simulink model "SIMU4INDIFullLoop"  (R2021a)
settings: Solver=VariableStepAuto  StartTime=0.0  StopTime=40  RelTol=1e-3
values from neighbouring files (symbols this model uses):
  Ahg2 = blkdiag(Ahg2, Ahcg)    [HinFSynINDIFullLoop.m]
  Ahs3 = blkdiag(Ahs3, Ahcs)    [HinFSynINDIFullLoop.m]
  Ahs7 = blkdiag(Ahs7, Ahcs)    [HinFSynINDIFullLoop.m]
  Amc = d2c(Amd,'tustin')    [HinFSynINDIFullLoop.m]
  Asc = d2c(Asd,'tustin')    [HinFSynINDIFullLoop.m]
  Bhg2 = blkdiag(Bhg2, Bhcg)    [HinFSynINDIFullLoop.m]
  Bhs3 = blkdiag(Bhs3, Bhcs)    [HinFSynINDIFullLoop.m]
  Bhs7 = blkdiag(Bhs7, Bhcs)    [HinFSynINDIFullLoop.m]
  Chg2 = blkdiag(Chg2, Chcg)    [HinFSynINDIFullLoop.m]
  Chs3 = blkdiag(Chs3, Chcs)    [HinFSynINDIFullLoop.m]
  Chs7 = blkdiag(Chs7, Chcs)    [HinFSynINDIFullLoop.m]
  Dhg2 = blkdiag(Dhg2, Dhcg)    [HinFSynINDIFullLoop.m]
  Dhs3 = blkdiag(Dhs3, Dhcs)    [HinFSynINDIFullLoop.m]
  Dhs7 = blkdiag(Dhs7, Dhcs)    [HinFSynINDIFullLoop.m]
  Gs = [-10.67  10.67  0     0     0     0 0 ... (first row only)    [HinFSynINDIFullLoop.m]
  Gs_inv = pinv(Gs)    [HinFSynINDIFullLoop.m]
  Kdg = diag([2.0; 1.8])    [HinFSynINDIFullLoop.m]
  Kds = [10; 18; 18]    [HinFSynINDIFullLoop.m]
  Kpg = blkdiag(Kposx.D,Kposz.D)    [HinFSynINDIFullLoop.m]
  Kps = [4.1089; 4.7304; 7.36]    [HinFSynINDIFullLoop.m]
settings Model: Creator=AutomZ2-RG02A02  LastModifiedBy=AutomZ2-RG02A02
settings SolverCC: AlgebraicLoopSolver=TrustRegion

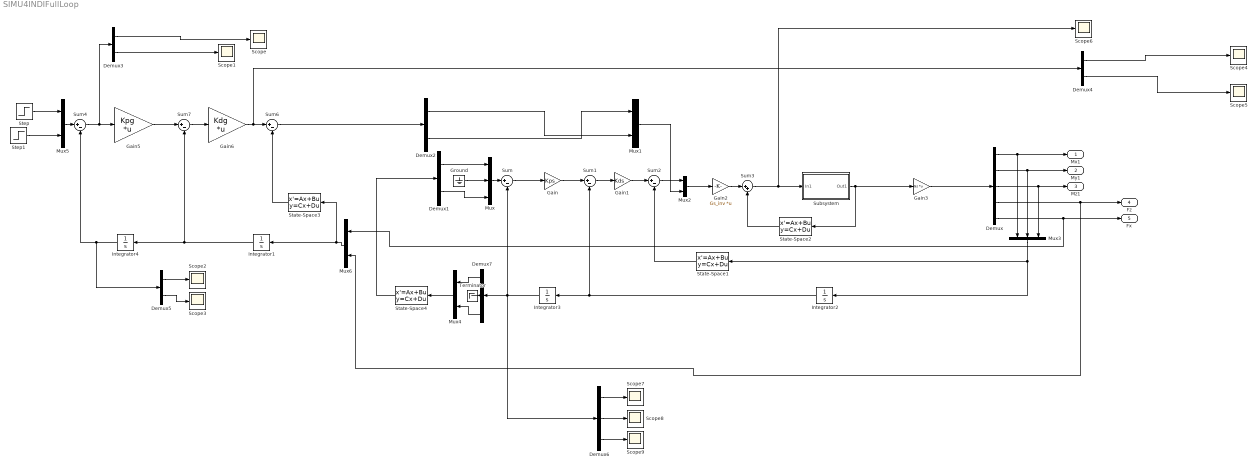
== system SIMU4INDIFullLoop ==
  Demux : Demux  Outputs=5
  Demux{1..5} (5 alike) : Demux  Outputs=2
  Demux6 : Demux  Outputs=3
  Demux7 : Demux  Outputs=3
  Gain : Gain  Gain=Kps
  Gain1 : Gain  Gain=Kds
  Gain2 : Gain  Gain=Gs_inv  Multiplication=Matrix(K*u)
  Gain3 : Gain  Gain=Gs  Multiplication=Matrix(K*u)
  Gain5 : Gain  Gain=Kpg  Multiplication=Matrix(K*u)
  Gain6 : Gain  Gain=Kdg  Multiplication=Matrix(K*u)
  Ground : Ground
  Integrator{1..4} (4 alike) : Integrator
  Mux : Mux  Inputs=3
  Mux{1,4..6} (4 alike) : Mux  Inputs=2
  Mux2 : Mux  Inputs=[3 2]
  Mux3 : Mux  Inputs=3
  Scope{,1..9} (10 alike) : Scope
  State-Space1 : StateSpace  A=Ahs3  B=Bhs3  C=Chs3  D=Dhs3  InitialCondition=0
  State-Space2 : StateSpace  A=Ahs7  B=Bhs7  C=Chs7  D=Dhs7  InitialCondition=0
  State-Space3 : StateSpace  A=Ahg2  B=Bhg2  C=Chg2  D=Dhg2  InitialCondition=0
  State-Space4 : StateSpace  A=Ahg2  B=Bhg2  C=Chg2  D=Dhg2  InitialCondition=0
  Step : Step  After=4  SampleTime=0
  Step1 : Step  Time=20  After=4  SampleTime=0
  Subsystem : Subsystem
  Sum{,1..2,4,6..7} (6 alike) : Sum  Inputs=|+-
  Sum3 : Sum  Inputs=|++
  Terminator : Terminator
  Mx1 : Outport
  My1 : Outport  Port=2
  Mz1 : Outport  Port=3
  Fz : Outport  Port=4
  Fx : Outport  Port=5
  wires:
  State-Space1/1 -> Sum2/2
  Subsystem/1(Out1) -> State-Space2/1, Gain3/1
  Mux/1 -> Sum/1
  Mux3/1 -> State-Space1/1, Integrator2/1
  Sum1/1 -> Gain1/1
  State-Space2/1 -> Sum3/2
  Integrator2/1 -> Sum1/2, Integrator3/1
  Sum2/1 -> Mux2/1
  Sum3/1 -> Scope6/1, Subsystem/1(In1)
  Mux1/1 -> Mux2/2
  Gain2/1 -> Sum3/1
  Demux/2 -> Mux3/2, My1/1
  Demux/3 -> Mz1/1, Mux3/3
  Gain/1 -> Sum1/1
  Mux2/1 -> Gain2/1
  Demux/1 -> Mux3/1, Mx1/1
  Sum/1 -> Gain/1
  Integrator3/1 -> Demux7/1, Sum/2, Demux6/1
  Gain1/1 -> Sum2/1
  Gain3/1 -> Demux/1
  Mux6/1 -> Integrator1/1, State-Space3/1
  Integrator1/1 -> Integrator4/1, Sum7/2
  Demux/5 -> Mux6/1, Fx/1
  Sum7/1 -> Gain6/1
  Step/1 -> Mux5/1
  Gain6/1 -> Demux4/1, Sum6/1
  Demux/4 -> Mux6/2, Fz/1
  Mux5/1 -> Sum4/1
  Gain5/1 -> Sum7/1
  Integrator4/1 -> Demux5/1, Sum4/2
  Sum6/1 -> Demux2/1
  State-Space3/1 -> Sum6/2
  Demux3/2 -> Scope1/1
  Sum4/1 -> Gain5/1, Demux3/1
  Demux3/1 -> Scope/1
  Demux4/2 -> Scope5/1
  Demux4/1 -> Scope4/1
  Step1/1 -> Mux5/2
  Demux5/1 -> Scope2/1
  Demux5/2 -> Scope3/1
  Demux2/1 -> Mux1/2
  Demux2/2 -> Mux1/1
  Demux6/1 -> Scope7/1
  Demux6/2 -> Scope8/1
  Demux6/3 -> Scope9/1
  Ground/1 -> Mux/2
  State-Space4/1 -> Demux1/1
  Demux7/2 -> Terminator/1
  Demux7/1 -> Mux4/1
  Demux7/3 -> Mux4/2
  Mux4/1 -> State-Space4/1
  Demux1/1 -> Mux/1
  Demux1/2 -> Mux/3

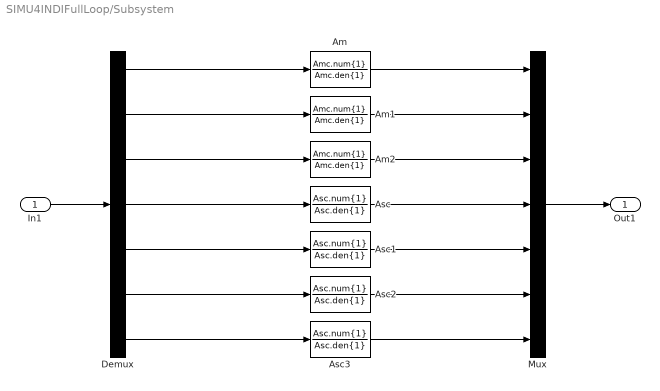
== system SIMU4INDIFullLoop/Subsystem ==
  In1 : Inport
  Am : TransferFcn  Numerator=Amc.num{1}  Denominator=Amc.den{1}
  Am1 : TransferFcn  Numerator=Amc.num{1}  Denominator=Amc.den{1}
  Am2 : TransferFcn  Numerator=Amc.num{1}  Denominator=Amc.den{1}
  Asc{,1..3} (4 alike) : TransferFcn  Numerator=Asc.num{1}  Denominator=Asc.den{1}
  Demux : Demux  Outputs=7
  Mux : Mux  Inputs=7
  Out1 : Outport
  wires:
  Demux/5 -> Asc1/1
  Asc/1 -> Mux/4
  Demux/4 -> Asc/1
  Asc1/1 -> Mux/5
  Asc2/1 -> Mux/6
  Demux/6 -> Asc2/1
  Asc3/1 -> Mux/7
  Demux/7 -> Asc3/1
  In1/1 -> Demux/1
  Mux/1 -> Out1/1
  Demux/1 -> Am/1
  Am/1 -> Mux/1
  Am1/1 -> Mux/2
  Demux/2 -> Am1/1
  Am2/1 -> Mux/3
  Demux/3 -> Am2/1
